simulink model "tutorial_ytgringo_Discretizacao_de_Controlador"  (R2020a)
settings: Solver=VariableStepAuto  StartTime=0.0  StopTime=10.0  RelTol=1e-3
values from neighbouring files (symbols this model uses):
  s = tf('s')    [Controlador_EE.m]    (also in Controlador_Ordem0_EE.m; Controlador_Ordem1_EE.m; Entendendo_controladores_BODE_Margin.m; FTMF_semcontrolador.m)
libraries: slctrlblks x4
settings Model: Creator=crist  LastModifiedBy=crist

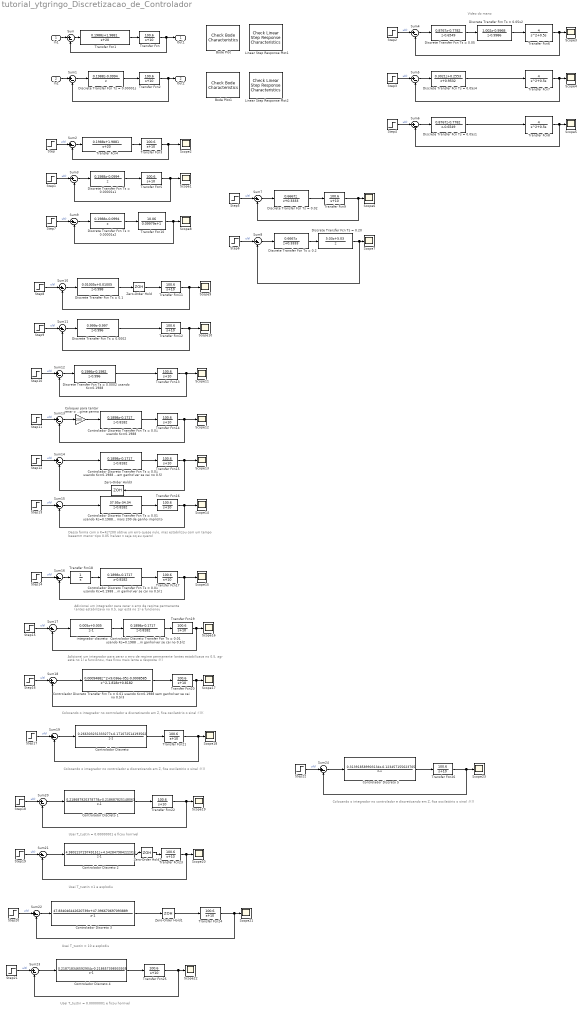
== system tutorial_ytgringo_Discretizacao_de_Controlador ==
  note: Adicionei um integrador para zerar o erro de regime permanente
      | (antes estabilizava no 0.5, agr está no 1) e funcionou
  note: Dessa forma com o K=Kc*200 obtive um erro quase nulo,
      | mas estabilizou com um tempo beeemm menor tipo 0.05 (talvez n seja oq eu quero)
  note: Video do mano
  note: Adicionei um integrador para zerar o erro de regime permanente
      | (antes estabilizava no 0.5, agr está no 1) e funcionou, mas ficou mais lenta a resposta :(((
  note: Colocando o integrador no controlador e discretizando em Z, fica oscilatório o sinal :((((
  note: Colocando o integrador no controlador e discretizando em Z, fica oscilatório o sinal :((((
  note: Usei T_tustin = 0.00000001 e ficou horrivel
  note: Usei T_tustin =1 e explodiu
  note: Usei T_tustin = 10 e explodiu
  note: Usei T_tustin = 0.00000001 e ficou horrivel
  note: Colocando o integrador no controlador e discretizando em Z, fica oscilatório o sinal :((((
  In1 : Inport
  In2 : Inport  Port=2
  Bode Plot : slctrlblks/Model Verification/Check Bode  Characteristics  InstantiateOnLoad=on  SaveOperatingPoints=off  LinearizationIOs={'/In1', 1, 'in', 'on', '';'/Transfer Fcn', 1, 'out', 'on', ''}  LinearizeAt=SnapshotTimes  SnapshotTimes=[0]  TriggerType=rising  SampleTime=auto  RateConversionMethod=zoh  PreWarpFreq=10  UseExactDelayModel=off  UseFullBlockNameLabels=off  UseBusSignalLabels=off  enabled=on  stopWhenAssertionFail=off  export=off  ViewDlgPos=[795 235 510 390]  OpenViewOnLoad=off  LaunchViewOnOpen=on  FrequencyUnits=rad/s  MagnitudeUnits=dB  PhaseUnits=deg  TimeUnits=seconds  EnableUpperBound=off  UpperBoundFrequencies=[]  UpperBoundMagnitudes=[]  EnableLowerBound=off  LowerBoundFrequencies=[]  LowerBoundMagnitudes=[]
  Bode Plot1 : slctrlblks/Model Verification/Check Bode  Characteristics  InstantiateOnLoad=on  SaveOperatingPoints=off  LinearizationIOs={'/In2', 1, 'in', 'on', '';'/Transfer Fcn2', 1, 'out', 'on', ''}  LinearizeAt=SnapshotTimes  SnapshotTimes=[0]  TriggerType=rising  SampleTime=auto  RateConversionMethod=zoh  PreWarpFreq=10  UseExactDelayModel=off  UseFullBlockNameLabels=off  UseBusSignalLabels=off  enabled=on  stopWhenAssertionFail=off  export=off  ViewDlgPos=[931 229 510 390]  OpenViewOnLoad=off  LaunchViewOnOpen=on  FrequencyUnits=rad/s  MagnitudeUnits=dB  PhaseUnits=deg  TimeUnits=seconds  EnableUpperBound=off  UpperBoundFrequencies=[]  UpperBoundMagnitudes=[]  EnableLowerBound=off  LowerBoundFrequencies=[]  LowerBoundMagnitudes=[]
  Coloquei para tentar zerar o erro de regime perma : Gain  Gain=200
  "Controlador Discreto " : DiscreteTransferFcn  Numerator=[0.266303231333277 -0.171072514193562]  Denominator=[1 -1]
  Controlador Discreto 1 : DiscreteTransferFcn  Numerator=[0.218687920378778 -0.218687825148061]  Denominator=[1 -1]
  Controlador Discreto 2 : DiscreteTransferFcn  Numerator=[4.980223729749151 4.542847984222311]  Denominator=[1 -1]
  Controlador Discreto 3 : DiscreteTransferFcn  Numerator=[47.834046442620739 47.396670697093889]  Denominator=[1 -1]
  Controlador Discreto 4 : DiscreteTransferFcn  Numerator=[0.218718346592904 -0.218657398933935]  Denominator=[1 -1]
  Controlador Discreto 5 : DiscreteTransferFcn  Numerator=[0.313918589903134 -0.123457155623705]  Denominator=[1 -1]
  Controlador Discreto Transfer Fcn Ts = 0.01 usando Kc=0.1988 : DiscreteTransferFcn  Numerator=[0.1898 -0.1717]  Denominator=[1 -0.8182]
  Controlador Discreto Transfer Fcn Ts = 0.01 usando Kc=0.1988 com mais 200 de ganho implicito : DiscreteTransferFcn  Numerator=[37.95 -34.34]  Denominator=[1 -0.8182]
  Controlador Discreto Transfer Fcn Ts = 0.01 usando Kc=0.1988 sem ganho(ver se cai no 0.5) : DiscreteTransferFcn  Numerator=[0.1898 -0.1717]  Denominator=[1 -0.8182]
  Controlador Discreto Transfer Fcn Ts = 0.01 usando Kc=0.1988 sem ganho(ver se cai no 0.5)1 : DiscreteTransferFcn  Numerator=[0.1898 -0.1717]  Denominator=[1 -0.8182]
  Controlador Discreto Transfer Fcn Ts = 0.01 usando Kc=0.1988 sem ganho(ver se cai no 0.5)2 : DiscreteTransferFcn  Numerator=[0.1898 -0.1717]  Denominator=[1 -0.8182]
  Controlador Discreto Transfer Fcn Ts = 0.01 usando Kc=0.1988 sem ganho(ver se cai no 0.5)3 : DiscreteTransferFcn  Numerator=[0.0009488 9.036e-05 -0.0008585]  Denominator=[1 -1.818 0.8182]
  Discrete Transfer Fcn Ts = 0.00001s : DiscreteTransferFcn  Numerator=[0.1988 -0.0994]  Denominator=[1 0]
  Discrete Transfer Fcn Ts = 0.00001s1 : DiscreteTransferFcn  Numerator=[0.1988 -0.0994]  Denominator=[1 0]
  Discrete Transfer Fcn Ts = 0.00001s2 : DiscreteTransferFcn  Numerator=[0.1988 -0.0994]  Denominator=[1 0]
  Discrete Transfer Fcn Ts = 0.0002 : DiscreteTransferFcn  Numerator=[0.999 -0.997]  Denominator=[1 -0.996]
  Discrete Transfer Fcn Ts = 0.0002 usando Kc=0.1988 : DiscreteTransferFcn  Numerator=[0.1986 -0.1982]  Denominator=[1 -0.996]
  Discrete Transfer Fcn Ts = 0.02 : DiscreteTransferFcn  Numerator=[0.6667 0]  Denominator=[1 0.3333]
  Discrete Transfer Fcn Ts = 0.05 : DiscreteTransferFcn  Numerator=[0.8767 -0.7782]  Denominator=[1 -0.6549]
  Discrete Transfer Fcn Ts = 0.05s1 : DiscreteTransferFcn  Numerator=[0.8767 -0.7782]  Denominator=[1 -0.6549]
  Discrete Transfer Fcn Ts = 0.05s2 : DiscreteTransferFcn  Numerator=[1.002 -0.9968]  Denominator=[1 -0.9986]
  Discrete Transfer Fcn Ts = 0.05s4 : DiscreteTransferFcn  Numerator=[0.3021 0.2553]  Denominator=[1 0.9532]
  Discrete Transfer Fcn Ts = 0.1 : DiscreteTransferFcn  Numerator=[0.01005 0.01005]  Denominator=[1 -0.998]
  Discrete Transfer Fcn Ts = 0.2 : DiscreteTransferFcn  Numerator=[0.6667 0]  Denominator=[1 0.3333]
  Discrete Transfer Fcn Ts = 0.20 : DiscreteTransferFcn  Numerator=[5.03 5.03]  Denominator=[1 0]
  Linear Step Response Plot1 : slctrlblks/Model Verification/Check Linear Step Response Characteristics  InstantiateOnLoad=on  SaveOperatingPoints=off  LinearizationIOs={'/In1', 1, 'in', 'off', '';'/Transfer Fcn', 1, 'out', 'off', ''}  LinearizeAt=SnapshotTimes  SnapshotTimes=[0]  TriggerType=rising  SampleTime=auto  RateConversionMethod=zoh  PreWarpFreq=10  UseExactDelayModel=off  UseFullBlockNameLabels=off  UseBusSignalLabels=off  enabled=on  stopWhenAssertionFail=off  export=off  ViewDlgPos=[591 211 546 385]  OpenViewOnLoad=off  LaunchViewOnOpen=on  FrequencyUnits=rad/s  MagnitudeUnits=dB  PhaseUnits=deg  TimeUnits=seconds  EnableStepResponseBound=off  FinalValue=[]  RiseTime=[]  PercentRise=[]  SettlingTime=[]  PercentSettling=[]  PercentOvershoot=[]  PercentUndershoot=[]
      settings: SourceProductBaseCode=SD  SaveToWorkspace=off  SaveName=sys
  Linear Step Response Plot2 : slctrlblks/Model Verification/Check Linear Step Response Characteristics  InstantiateOnLoad=on  SaveOperatingPoints=off  LinearizationIOs={'/In2', 1, 'in', 'off', '';'/Transfer Fcn2', 1, 'out', 'off', ''}  LinearizeAt=SnapshotTimes  SnapshotTimes=[0]  TriggerType=rising  SampleTime=auto  RateConversionMethod=zoh  PreWarpFreq=10  UseExactDelayModel=off  UseFullBlockNameLabels=off  UseBusSignalLabels=off  enabled=on  stopWhenAssertionFail=off  export=off  ViewDlgPos=[449 252 510 390]  OpenViewOnLoad=off  LaunchViewOnOpen=on  FrequencyUnits=rad/s  MagnitudeUnits=dB  PhaseUnits=deg  TimeUnits=seconds  EnableStepResponseBound=off  FinalValue=[]  RiseTime=[]  PercentRise=[]  SettlingTime=[]  PercentSettling=[]  PercentOvershoot=[]  PercentUndershoot=[]
      settings: SourceProductBaseCode=SD  SaveToWorkspace=off  SaveName=sys
  Scope{1..23} (23 alike) : Scope
  Step{,1..22} (23 alike) : Step  SampleTime=0
  Sum{,1..24} (25 alike) : Sum  Inputs=|+-
  Transfer Fcn{,2..3,5,9,11..17,19..26} (20 alike) : TransferFcn  Numerator=[100.6]  Denominator=[1 10]
  Transfer Fcn1 : TransferFcn  Numerator=[0.1988 1.9881]  Denominator=[1 20]
  Transfer Fcn10 : TransferFcn  Numerator=[10.06]  Denominator=[0.09979 1]
  Transfer Fcn18 : TransferFcn  Denominator=[1 0]
  Transfer Fcn4 : TransferFcn  Numerator=[0.1988 1.9881]  Denominator=[1 20]
  Transfer Fcn6 : TransferFcn  Numerator=[4]  Denominator=[1 0.5 0]
  Transfer Fcn7 : TransferFcn  Numerator=[4]  Denominator=[1 0.5 0]
  Transfer Fcn8 : TransferFcn  Numerator=[4]  Denominator=[1 0.5 0]
  Zero-Order Hold : ZeroOrderHold  SampleTime=0.0002
  Zero-Order Hold1 : ZeroOrderHold  SampleTime=10
  Zero-Order Hold2 : ZeroOrderHold
  Zero-Order Hold3 : ZeroOrderHold  SampleTime=0.01
  integrador discreto : DiscreteTransferFcn  Numerator=[0.005 0.005]  Denominator=[1 -1]
  Out1 : Outport
  Out2 : Outport  Port=2
  wires:
  Transfer Fcn1/1 -> Transfer Fcn/1
  Transfer Fcn/1 -> Sum/2, Out1/1
  In1/1 -> Sum/1
  Transfer Fcn2/1 -> Sum1/2, Out2/1
  In2/1 -> Sum1/1
  Discrete Transfer Fcn Ts = 0.00001s/1 -> Transfer Fcn2/1
  Sum1/1 -> Discrete Transfer Fcn Ts = 0.00001s/1
  Sum/1 -> Transfer Fcn1/1
  Sum2/1 -> Transfer Fcn4/1
  Transfer Fcn3/1 -> Scope2/1, Sum2/2
  Transfer Fcn4/1 -> Transfer Fcn3/1
  Step/1 -> Sum2/1  "u(t)"
  Transfer Fcn5/1 -> Scope1/1, Sum3/2
  Sum3/1 -> Discrete Transfer Fcn Ts = 0.00001s1/1
  Discrete Transfer Fcn Ts = 0.00001s1/1 -> Transfer Fcn5/1
  Step1/1 -> Sum3/1  "u(t)"
  Step2/1 -> Sum4/1  "u(t)"
  Transfer Fcn6/1 -> Scope3/1, Sum4/2
  Sum4/1 -> Discrete Transfer Fcn Ts = 0.05/1
  Discrete Transfer Fcn Ts = 0.05/1 -> Discrete Transfer Fcn Ts = 0.05s2/1
  Discrete Transfer Fcn Ts = 0.05s2/1 -> Transfer Fcn6/1
  Transfer Fcn7/1 -> Scope4/1, Sum5/2
  Step3/1 -> Sum5/1  "u(t)"
  Sum5/1 -> Discrete Transfer Fcn Ts = 0.05s4/1
  Discrete Transfer Fcn Ts = 0.05s4/1 -> Transfer Fcn7/1
  Discrete Transfer Fcn Ts = 0.05s1/1 -> Transfer Fcn8/1
  Step4/1 -> Sum6/1  "u(t)"
  Sum6/1 -> Discrete Transfer Fcn Ts = 0.05s1/1
  Transfer Fcn8/1 -> Scope5/1, Sum6/2
  Step5/1 -> Sum7/1  "u(t)"
  Discrete Transfer Fcn Ts = 0.02/1 -> Transfer Fcn9/1
  Transfer Fcn9/1 -> Scope6/1, Sum7/2
  Sum7/1 -> Discrete Transfer Fcn Ts = 0.02/1
  Discrete Transfer Fcn Ts = 0.2/1 -> Discrete Transfer Fcn Ts = 0.20/1
  Discrete Transfer Fcn Ts = 0.20/1 -> Scope7/1, Sum8/2
  Sum8/1 -> Discrete Transfer Fcn Ts = 0.2/1
  Step6/1 -> Sum8/1  "u(t)"
  Step7/1 -> Sum9/1  "u(t)"
  Discrete Transfer Fcn Ts = 0.00001s2/1 -> Transfer Fcn10/1
  Transfer Fcn10/1 -> Scope8/1, Sum9/2
  Sum9/1 -> Discrete Transfer Fcn Ts = 0.00001s2/1
  Step8/1 -> Sum10/1  "u(t)"
  Transfer Fcn11/1 -> Scope9/1, Sum10/2
  Sum10/1 -> Discrete Transfer Fcn Ts = 0.1/1
  Zero-Order Hold/1 -> Transfer Fcn11/1
  Discrete Transfer Fcn Ts = 0.1/1 -> Zero-Order Hold/1
  Transfer Fcn12/1 -> Scope10/1, Sum11/2
  Sum11/1 -> Discrete Transfer Fcn Ts = 0.0002/1
  Step9/1 -> Sum11/1  "u(t)"
  Discrete Transfer Fcn Ts = 0.0002/1 -> Transfer Fcn12/1
  Discrete Transfer Fcn Ts = 0.0002 usando Kc=0.1988/1 -> Transfer Fcn13/1
  Transfer Fcn13/1 -> Scope11/1, Sum12/2
  Step10/1 -> Sum12/1  "u(t)"
  Sum12/1 -> Discrete Transfer Fcn Ts = 0.0002 usando Kc=0.1988/1
  Sum13/1 -> Coloquei para tentar zerar o erro de regime perma/1
  Transfer Fcn14/1 -> Scope12/1, Sum13/2
  Step11/1 -> Sum13/1  "u(t)"
  Controlador Discreto Transfer Fcn Ts = 0.01 usando Kc=0.1988/1 -> Transfer Fcn14/1
  Coloquei para tentar zerar o erro de regime perma/1 -> Controlador Discreto Transfer Fcn Ts = 0.01 usando Kc=0.1988/1
  Transfer Fcn15/1 -> Scope13/1, Zero-Order Hold3/1
  Sum14/1 -> Controlador Discreto Transfer Fcn Ts = 0.01 usando Kc=0.1988 sem ganho(ver se cai no 0.5)/1
  Controlador Discreto Transfer Fcn Ts = 0.01 usando Kc=0.1988 sem ganho(ver se cai no 0.5)/1 -> Transfer Fcn15/1
  Step12/1 -> Sum14/1  "u(t)"
  Step13/1 -> Sum15/1  "u(t)"
  Transfer Fcn16/1 -> Scope14/1, Sum15/2
  Controlador Discreto Transfer Fcn Ts = 0.01 usando Kc=0.1988 com mais 200 de ganho implicito/1 -> Transfer Fcn16/1
  Sum15/1 -> Controlador Discreto Transfer Fcn Ts = 0.01 usando Kc=0.1988 com mais 200 de ganho implicito/1
  Step14/1 -> Sum16/1  "u(t)"
  Transfer Fcn17/1 -> Scope15/1, Sum16/2
  Controlador Discreto Transfer Fcn Ts = 0.01 usando Kc=0.1988 sem ganho(ver se cai no 0.5)1/1 -> Transfer Fcn17/1
  Sum16/1 -> Transfer Fcn18/1
  Transfer Fcn18/1 -> Controlador Discreto Transfer Fcn Ts = 0.01 usando Kc=0.1988 sem ganho(ver se cai no 0.5)1/1
  Sum17/1 -> integrador discreto/1
  Transfer Fcn19/1 -> Scope16/1, Sum17/2
  Controlador Discreto Transfer Fcn Ts = 0.01 usando Kc=0.1988 sem ganho(ver se cai no 0.5)2/1 -> Transfer Fcn19/1
  integrador discreto/1 -> Controlador Discreto Transfer Fcn Ts = 0.01 usando Kc=0.1988 sem ganho(ver se cai no 0.5)2/1
  Step15/1 -> Sum17/1  "u(t)"
  Step16/1 -> Sum18/1  "u(t)"
  Controlador Discreto Transfer Fcn Ts = 0.01 usando Kc=0.1988 sem ganho(ver se cai no 0.5)3/1 -> Transfer Fcn20/1
  Transfer Fcn20/1 -> Scope17/1, Sum18/2
  Sum18/1 -> Controlador Discreto Transfer Fcn Ts = 0.01 usando Kc=0.1988 sem ganho(ver se cai no 0.5)3/1
  Transfer Fcn21/1 -> Scope18/1, Sum19/2
  Step17/1 -> Sum19/1  "u(t)"
  "Controlador Discreto "/1 -> Transfer Fcn21/1
  Sum19/1 -> "Controlador Discreto "/1
  Controlador Discreto 1/1 -> Transfer Fcn22/1
  Step18/1 -> Sum20/1  "u(t)"
  Sum20/1 -> Controlador Discreto 1/1
  Transfer Fcn22/1 -> Scope19/1, Sum20/2
  Step19/1 -> Sum21/1  "u(t)"
  Sum21/1 -> Controlador Discreto 2/1
  Transfer Fcn23/1 -> Scope20/1, Sum21/2
  Controlador Discreto 2/1 -> Zero-Order Hold2/1
  Step20/1 -> Sum22/1  "u(t)"
  Sum22/1 -> Controlador Discreto 3/1
  Transfer Fcn24/1 -> Scope21/1, Sum22/2
  Controlador Discreto 3/1 -> Zero-Order Hold1/1
  Zero-Order Hold1/1 -> Transfer Fcn24/1
  Zero-Order Hold2/1 -> Transfer Fcn23/1
  Step21/1 -> Sum23/1  "u(t)"
  Sum23/1 -> Controlador Discreto 4/1
  Transfer Fcn25/1 -> Scope22/1, Sum23/2
  Controlador Discreto 4/1 -> Transfer Fcn25/1
  Controlador Discreto 5/1 -> Transfer Fcn26/1
  Transfer Fcn26/1 -> Scope23/1, Sum24/2
  Step22/1 -> Sum24/1  "u(t)"
  Sum24/1 -> Controlador Discreto 5/1
  Zero-Order Hold3/1 -> Sum14/2
